simulink model "model_fm2"  (R2022a)
settings: Solver=FixedStepDiscrete  StartTime=0.0  StopTime=inf  RelTol=1e-3
libraries: commdigbbndfm2 x2, commchan3 x1, commrandsrc3 x1, commsink2 x1, commutil2 x1
settings Model: Creator=D.mon  LastModifiedBy=D.mon
settings ModelReferenceCC: EnableRefExpFcnMdlSchedulingChecks=off
settings RTWCC: Description=Generic Real-Time Target  GPUComputeCapability=5.0
settings ConfigComp: CovBoundaryAbsTol=1.0e-5

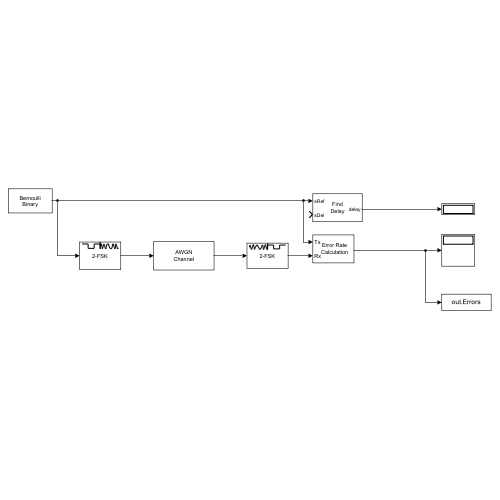
[thumbnail: Simulink's stored preview of the top-level diagram]
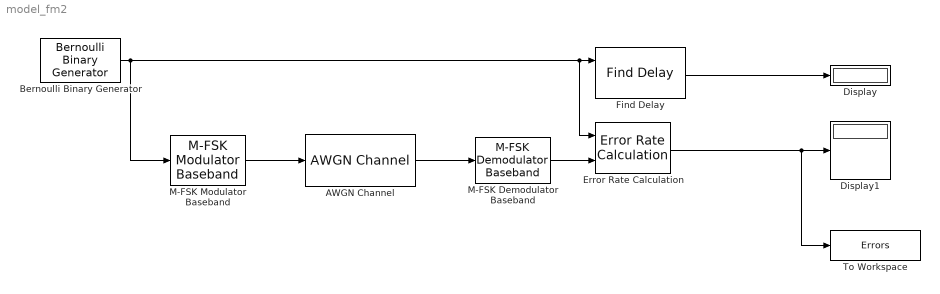
== system model_fm2 ==
  AWGN Channel : commchan3/AWGN Channel  InputProcessing=Columns as channels (frame based)  noiseMode="Signal to noise ratio  (SNR)"  EbNodB=EbPerNo  EsNodB=10  SNRdB=10  bitsPerSym=1  Ps=1  Tsym=1  variance=1  seed=67
  Bernoulli Binary Generator : commrandsrc3/Bernoulli Binary Generator  ProbabilityOfZero=0.5  SeedSource=Auto  Seed=0  SampleTime=1e-3  SamplesPerFrame=1000  OutputDataType=double  SimulateUsing=Interpreted execution
  Display : Display
  Display1 : Display
  Error Rate Calculation : commsink2/Error Rate Calculation  N=0  st_delay=0  cp_mode=Entire frame  subframe=[]  PMode=Port  WsName=ErrorVec  RsMode2=off  stop=on  numErr=100  maxBits=1e6
  Find Delay : commutil2/Find Delay  corrLength=200  chgSigOP=off  stopUpdate=off  numConstDelay=3
  M-FSK Demodulator Baseband : commdigbbndfm2/M-FSK Demodulator Baseband  M=2  OutType=Integer  Dec=Gray  freqSep=2e3  numSamp=16  RateOptions=Enforce single-rate processing  outDataType=double
  M-FSK Modulator Baseband : commdigbbndfm2/M-FSK Modulator Baseband  M=2  InType=Integer  Enc=Gray  freqSep=2e3  phaseType=Continuous  numSamp=16  RateOptions=Enforce single-rate processing  outDataType=double
  To Workspace : ToWorkspace  VariableName=Errors  SampleTime=-1
      settings: MaxDataPoints=1
  wires:
  Error Rate Calculation/1 -> To Workspace/1, Display1/1
  Find Delay/1 -> Display/1
  Bernoulli Binary Generator/1 -> M-FSK Modulator Baseband/1, Error Rate Calculation/1, Find Delay/1
  M-FSK Modulator Baseband/1 -> AWGN Channel/1
  M-FSK Demodulator Baseband/1 -> Error Rate Calculation/2
  AWGN Channel/1 -> M-FSK Demodulator Baseband/1
